simulink model "chap4_3"  (R2021b)
settings: Solver=VariableStepAuto  StartTime=0.0  StopTime=10.0  RelTol=1e-3
libraries: fuzblock x1
settings Model: Creator=16690  LastModifiedBy=16690

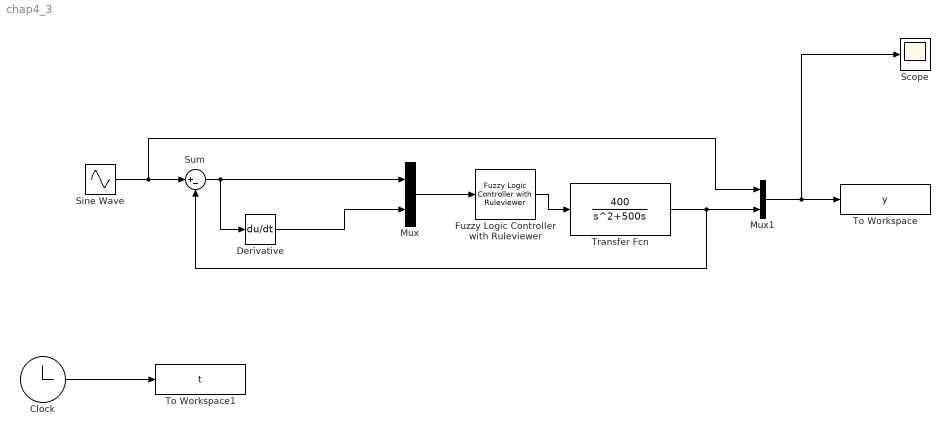
== system chap4_3 ==
  Clock : Clock
  Derivative : Derivative
  Fuzzy Logic Controller with Ruleviewer : fuzblock/Fuzzy Logic  Controller  with Ruleviewer  fismatrix=a2  Ts=2
  Mux : Mux  Inputs=2
  Mux1 : Mux  Inputs=2
  Scope : Scope
  Sine Wave : Sin  Amplitude=0.5  Frequency=10  SampleTime=0
  Sum : Sum  Inputs=|+-
  To Workspace : ToWorkspace  VariableName=y  SaveFormat=Timeseries  SampleTime=-1
  To Workspace1 : ToWorkspace  VariableName=t  SaveFormat=Timeseries  SampleTime=-1
  Transfer Fcn : TransferFcn  Numerator=[400]  Denominator=[1 500 0]
  wires:
  Sine Wave/1 -> Mux1/1, Sum/1
  Sum/1 -> Derivative/1, Mux/1
  Derivative/1 -> Mux/2
  Mux/1 -> Fuzzy Logic Controller with Ruleviewer/1
  Fuzzy Logic Controller with Ruleviewer/1 -> Transfer Fcn/1
  Mux1/1 -> Scope/1, To Workspace/1
  Transfer Fcn/1 -> Sum/2, Mux1/2
  Clock/1 -> To Workspace1/1
